simulink model "Subsystem"  (R2020b)
settings: Solver=FixedStepDiscrete  StartTime=0.0  StopTime=10.0  FixedStep=0.1  RelTol=1e-3
settings Model: Creator=Diwakar Reddy  LastModifiedBy=Diwakar Reddy
settings DataIOCC: SaveOutput=off  SaveTime=off

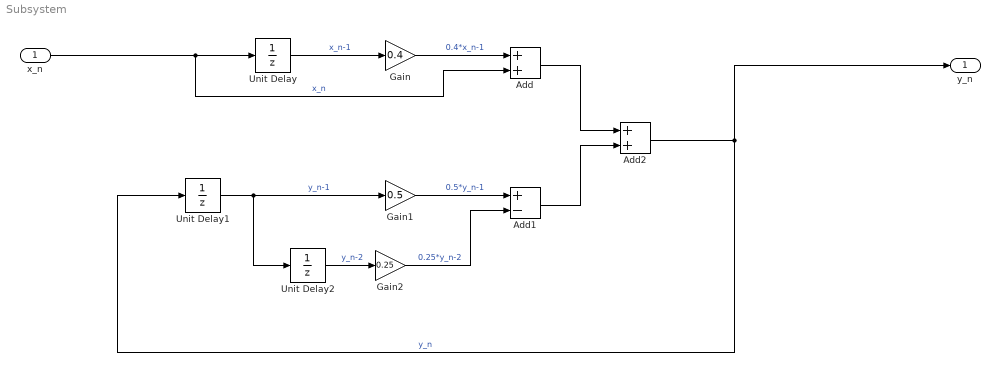
== system Subsystem ==
  x_n : Inport  OutDataTypeStr=double  PortDimensions=1  SampleTime=0
  Add : Sum
  Add1 : Sum  Inputs=+-
  Add2 : Sum
  Gain : Gain  Gain=0.4
  Gain1 : Gain  Gain=0.5
  Gain2 : Gain  Gain=0.25
  Unit Delay : UnitDelay  SampleTime=-1  HasFrameUpgradeWarning=on
  Unit Delay1 : UnitDelay  SampleTime=-1  HasFrameUpgradeWarning=on
  Unit Delay2 : UnitDelay  SampleTime=-1  HasFrameUpgradeWarning=on
  y_n : Outport  OutDataTypeStr=double  PortDimensions=1  SampleTime=0
  wires:
  Unit Delay/1 -> Gain/1  "x_n-1"
  Add2/1 -> Unit Delay1/1, y_n/1  "y_n"
  Add1/1 -> Add2/2
  Unit Delay1/1 -> Gain1/1, Unit Delay2/1  "y_n-1"
  x_n/1 -> Unit Delay/1, Add/2  "x_n"
  Gain2/1 -> Add1/2  "0.25*y_n-2"
  Gain/1 -> Add/1  "0.4*x_n-1"
  Gain1/1 -> Add1/1  "0.5*y_n-1"
  Add/1 -> Add2/1
  Unit Delay2/1 -> Gain2/1  "y_n-2"
